simulink model "model_15a"  (R2020a)
settings: Solver=ode3  StartTime=0.0  StopTime=100  FixedStep=Ts  RelTol=1e-3
undefined symbols (not defined in the file): A, B, C, F, R
settings Model: Creator=bosold  LastModifiedBy=bosold
settings OptimizationCC: LifeSpan=inf
settings DebuggingCC: SFExecutionAtInitializationDiag=none  ArithmeticOperatorsInVariantConditions=warning
settings HardwareCC: ProdBitPerSizeT=32  ProdBitPerPtrDiffT=32  ProdWordSize=32  ProdHWDeviceType=Specified
settings SFSimCC: CustomCodeUndefinedFunction=UseInterfaceOnly
settings CodeAppCC: StateflowObjectComments=on

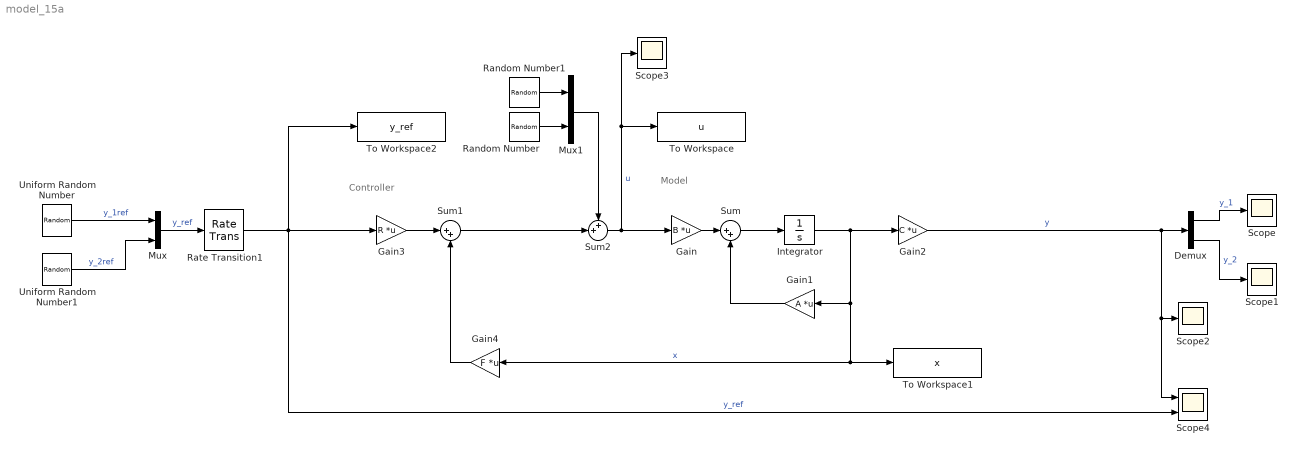
== system model_15a ==
  note: Controller
  note: Model
  Demux : Demux  Outputs=2
  Gain : Gain  Gain=B  Multiplication=Matrix(K*u)
  Gain1 : Gain  Gain=A  Multiplication=Matrix(K*u)
  Gain2 : Gain  Gain=C  Multiplication=Matrix(K*u)
  Gain3 : Gain  Gain=R  Multiplication=Matrix(K*u)
  Gain4 : Gain  Gain=F  Multiplication=Matrix(K*u)
  Integrator : Integrator
  Mux : Mux  Inputs=2
  Mux1 : Mux  Inputs=2
  Random Number : RandomNumber  Seed=2  SampleTime=0.1
  Random Number1 : RandomNumber  Variance=3  SampleTime=0.1
  Rate Transition1 : RateTransition  OutPortSampleTime=Ts
  Scope{,1..3} (4 alike) : Scope
  Scope4 : Scope  NumInputPorts=2
  Sum : Sum  Inputs=|++
  Sum1 : Sum  Inputs=|++
  Sum2 : Sum  Inputs=++|
  To Workspace : ToWorkspace  VariableName=u  SaveFormat=Timeseries  SampleTime=-1
  To Workspace1 : ToWorkspace  VariableName=x  SaveFormat=Timeseries  SampleTime=-1
  To Workspace2 : ToWorkspace  VariableName=y_ref  SaveFormat=Timeseries  SampleTime=-1
  Uniform Random Number : UniformRandomNumber  Minimum=-10  Maximum=10  SampleTime=10
  Uniform Random Number1 : UniformRandomNumber  Minimum=-10  Maximum=10  Seed=1  SampleTime=10
  wires:
  Sum/1 -> Integrator/1
  Gain/1 -> Sum/1
  Integrator/1 -> Gain2/1, To Workspace1/1, Gain4/1, Gain1/1  "x"
  Gain1/1 -> Sum/2
  Rate Transition1/1 -> To Workspace2/1, Scope4/2, Gain3/1  "y_ref"
  Uniform Random Number/1 -> Mux/1  "y_1ref"
  Uniform Random Number1/1 -> Mux/2  "y_2ref"
  Gain2/1 -> Scope4/1, Scope2/1, Demux/1  "y"
  Demux/1 -> Scope/1  "y_1"
  Demux/2 -> Scope1/1  "y_2"
  Sum1/1 -> Sum2/2
  Gain3/1 -> Sum1/1
  Gain4/1 -> Sum1/2
  Sum2/1 -> Scope3/1, To Workspace/1, Gain/1  "u"
  Mux1/1 -> Sum2/1
  Random Number/1 -> Mux1/2
  Random Number1/1 -> Mux1/1
  Mux/1 -> Rate Transition1/1  "y_ref"
